simulink model "main__"  (R2013b)
settings: Solver=ode3  StartTime=0.0  StopTime=inf  RelTol=1e-3
undefined symbols (not defined in the file): DiscIntNeverNeededParam, st_, Standard_Devices, UDP_Protocol
libraries: rtwinlib x4
settings Model: SimulationMode=external  ExtModeTrigDuration=1000001  BufferReuse=off  Creator=Nabeel  LastModifiedBy=Nabeel Ahmad
settings SolverCC: AutoInsertRateTranBlk=on
settings DataIOCC: LimitDataPoints=off  SaveOutput=off  SaveTime=off
settings OptimizationCC: OptimizeBlockIOStorage=off  BufferReuse=off  ExpressionFolding=off  LocalBlockOutputs=off
settings DebuggingCC: StateNameClashWarn=warning
settings HardwareCC: ProdIntDivRoundTo=Zero  ProdEndianess=LittleEndian  ProdHWDeviceType=Generic->32-bit x86 compatible
settings RTWCC: SystemTargetFile=rtwin.tlc  TemplateMakefile=rtwin.tmf  Description=Real-Time Windows Target  ProcessScript=rtwin_make_rtw_hook  RTWCompilerOptimization=On
settings CodeAppCC: MaxIdLength=95
settings RTWinTargetCC: TargetLibSuffix=_rtwin.lib  TargetPreCompLibLocation=C:\Program Files\MATLAB\R2013b\toolbox\rtw\targets\rtwin\lib\win64  CodeReplacementLibrary=ANSI_C  RTWinDir=C:/PROGRA~1/MATLAB/R2013b/toolbox/rtw/targets/rtwin  TargetArch=win64

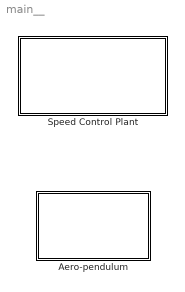
== system main__ ==
  Aero-pendulum : Subsystem
  Speed Control Plant : Subsystem

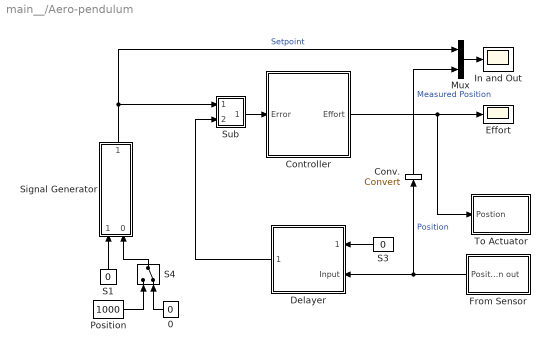
== system main__/Aero-pendulum ==
  0 : Constant  Value=0
  Controller : Subsystem
  Conv. : DataTypeConversion
  Delayer : Subsystem
  Effort : Scope
      settings: TimeRange=100  YMin=33.5  YMax=33.5  SaveName=ScopeData4
  From Sensor : Subsystem
  In and Out : Scope
      settings: ShowLegends=on  TimeRange=40  YMin=-90  YMax=90  SaveName=ScopeData5
  Mux : Mux  Inputs=2
  Position : Constant  Value=1000
  S1 : Constant  Value=0
  S3 : Constant  Value=0
  S4 : ManualSwitch  CurrentSetting=0
  Signal Generator : Subsystem
  Sub : Subsystem
  To Actuator : Subsystem
  wires:
  Delayer/1(Output) -> Sub/2(F)
  Controller/1(Effort) -> To Actuator/1(Postion), Effort/1
  Signal Generator/1(Set Point) -> Mux/1, Sub/1(S)  "Setpoint"
  S3/1 -> Delayer/1(Setting)
  Conv./1 -> Mux/2  "Measured Position"
  Mux/1 -> In and Out/1
  Sub/1(E) -> Controller/1(Error)
  From Sensor/1(Position out) -> Delayer/2(Input), Conv./1  "Position"
  Position/1 -> S4/1
  S4/1 -> Signal Generator/2(0)
  0/1 -> S4/2
  S1/1 -> Signal Generator/1(Setting)

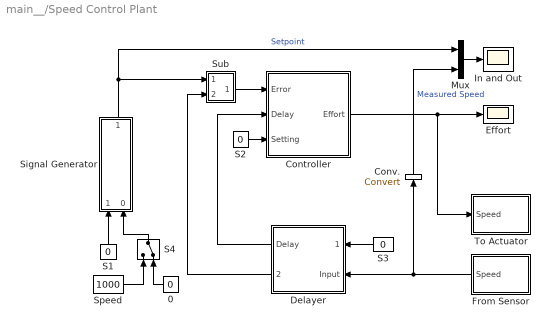
== system main__/Speed Control Plant ==
  0 : Constant  Value=0
  Controller : Subsystem
  Conv. : DataTypeConversion
  Delayer : Subsystem
  Effort : Scope
      settings: TimeRange=100  YMin=-2136.75  YMax=-1933.25
  From Sensor : Subsystem
  In and Out : Scope
      settings: ShowLegends=on  TimeRange=60  YMin=-500  YMax=2100
  Mux : Mux  Inputs=2
  S1 : Constant  Value=0
  S2 : Constant  Value=0
  S3 : Constant  Value=0
  S4 : ManualSwitch  CurrentSetting=0
  Signal Generator : Subsystem
  Speed : Constant  Value=1000
  Sub : Subsystem
  To Actuator : Subsystem
  wires:
  Conv./1 -> Mux/2  "Measured Speed"
  Controller/1(Effort) -> To Actuator/1(Speed), Effort/1
  S2/1 -> Controller/3(Setting)
  Speed/1 -> S4/1
  S4/1 -> Signal Generator/2(0)
  0/1 -> S4/2
  From Sensor/1(Speed) -> Delayer/2(Input), Conv./1
  Signal Generator/1(Set Point) -> Sub/1(S), Mux/1  "Setpoint"
  S1/1 -> Signal Generator/1(Setting)
  Mux/1 -> In and Out/1
  Sub/1(E) -> Controller/1(Error)
  Delayer/1(Delay) -> Controller/2(Delay)
  S3/1 -> Delayer/1(Setting)
  Delayer/2(Output) -> Sub/2(F)

== system main__/Aero-pendulum/Controller ==
  Error : Inport
  I : Constant  Value=.4
  P : Constant  Value=.15
  PI Controller : Subsystem
  Trigger : Constant  Value=0
  Effort : Outport
  wires:
  Trigger/1 -> PI Controller/4(Reset)
  I/1 -> PI Controller/3(I)
  P/1 -> PI Controller/2(P)
  Error/1 -> PI Controller/1(Error)
  PI Controller/1(Effort) -> Effort/1  "Effort"

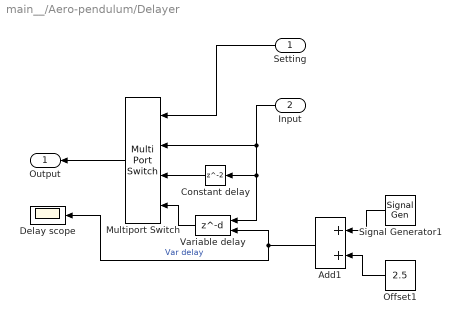
== system main__/Aero-pendulum/Delayer ==
  Setting : Inport
  Input : Inport  Port=2
  Add1 : Sum  OutDataTypeStr=uint8
  Constant delay : Delay  InitialCondition=0  SampleTime=st_
  Delay scope : Scope
      settings: TimeRange=100  YMin=0  SaveName=ScopeData2
  Multiport Switch : MultiPortSwitch  DataPortOrder=Zero-based contiguous
  Offset1 : Constant  Value=2.5
  Signal Generator1 : SignalGenerator  WaveForm=sawtooth  Amplitude=2.5  Frequency=.01
  Variable delay : Delay  DelayLengthSource=Input port  InitialCondition=0  SampleTime=st_
      settings: InputPortMap=u0,p1
  Output : Outport
  wires:
  Setting/1 -> Multiport Switch/1
  Variable delay/1 -> Multiport Switch/4
  Multiport Switch/1 -> Output/1
  Signal Generator1/1 -> Add1/1
  Add1/1 -> Delay scope/1, Variable delay/2  "Var delay"
  Offset1/1 -> Add1/2
  Input/1 -> Multiport Switch/2, Variable delay/1, Constant delay/1
  Constant delay/1 -> Multiport Switch/3

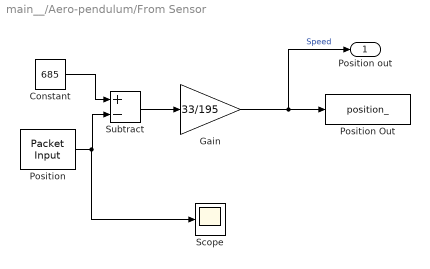
== system main__/Aero-pendulum/From Sensor ==
  Constant : Constant  Value=685
  Gain : Gain  Gain=33/195
  Position : rtwinlib/Packet Input  SampleTime=st_  MaxMissedTicks=10  ShowMissedTicks=off  YieldWhenWaiting=off  DrvName=Standard_Devices/UDP_Protocol  DrvAddress=12349  DrvOptions=[3232235531 43210]  PacketSize=2  DataTypes='int16'  ShowReady=off  ShowError=off  PacketID=1  ByteOrder=1  ShowTimestamp=off
      settings: AttributesFormatString=Standard Devices\nUDP Protocol [303Dh]
  Position Out : ToWorkspace  VariableName=position_  SampleTime=st_  SaveFormat=Structure With Time
  Scope : Scope
      settings: YMin=0  YMax=850  SaveName=ScopeData3
  Subtract : Sum  Inputs=+-
  Position out : Outport
  wires:
  Gain/1 -> Position Out/1, Position out/1  "Speed"
  Subtract/1 -> Gain/1
  Constant/1 -> Subtract/1
  Position/1 -> Scope/1, Subtract/2

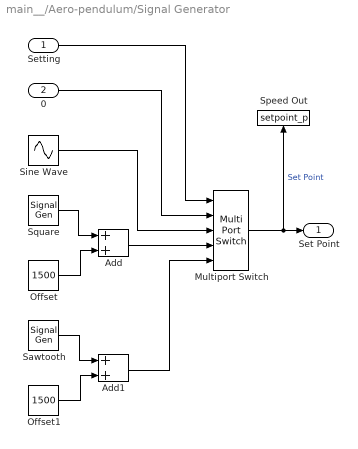
== system main__/Aero-pendulum/Signal Generator ==
  Setting : Inport
  0 : Inport  Port=2
  Add : Sum
  Add1 : Sum
  Multiport Switch : MultiPortSwitch  DataPortOrder=Zero-based contiguous  Inputs=4
  Offset : Constant  Value=1500
  Offset1 : Constant  Value=1500
  Sawtooth : SignalGenerator  WaveForm=square  Amplitude=400  Frequency=.2
  Sine Wave : Sin  Amplitude=7  Bias=15  Frequency=.2  SampleTime=0
  Speed Out : ToWorkspace  VariableName=setpoint_p  SampleTime=st_  SaveFormat=Structure With Time
  Square : SignalGenerator  WaveForm=sawtooth  Amplitude=400  Frequency=.2
  Set Point : Outport
  wires:
  Offset/1 -> Add/2
  Multiport Switch/1 -> Speed Out/1, Set Point/1  "Set Point"
  Setting/1 -> Multiport Switch/1
  Add/1 -> Multiport Switch/4
  0/1 -> Multiport Switch/2
  Sine Wave/1 -> Multiport Switch/3
  Square/1 -> Add/1
  Offset1/1 -> Add1/2
  Add1/1 -> Multiport Switch/5
  Sawtooth/1 -> Add1/1

== system main__/Aero-pendulum/Sub ==
  S : Inport
  F : Inport  Port=2
  Constant : Constant  Value=0
  Manual Switch : ManualSwitch  CurrentSetting=0
  Sum : Sum  Inputs=|+-
  E : Outport
  wires:
  Sum/1 -> E/1
  S/1 -> Sum/1
  Constant/1 -> Manual Switch/1
  F/1 -> Manual Switch/2
  Manual Switch/1 -> Sum/2

== system main__/Aero-pendulum/To Actuator ==
  Postion : Inport
  Position Out : ToWorkspace  VariableName=effort_p  SampleTime=st_  SaveFormat=Structure With Time
  Position Set Point : rtwinlib/Packet Output  SampleTime=st_  MaxMissedTicks=10  ShowMissedTicks=off  YieldWhenWaiting=off  DrvName=Standard_Devices/UDP_Protocol  DrvAddress=12351  DrvOptions=[3232235531 43210]  PacketSize=2  DataTypes='int16'  ShowReady=off  ShowError=off  PacketID=1  ByteOrder=1  InitialValue=[]  FinalValue=[]
      settings: AttributesFormatString=Standard Devices\nUDP Protocol [303Fh]
  Position to PWM duty : Gain  Gain=255/33
  wires:
  Postion/1 -> Position to PWM duty/1, Position Out/1
  Position to PWM duty/1 -> Position Set Point/1

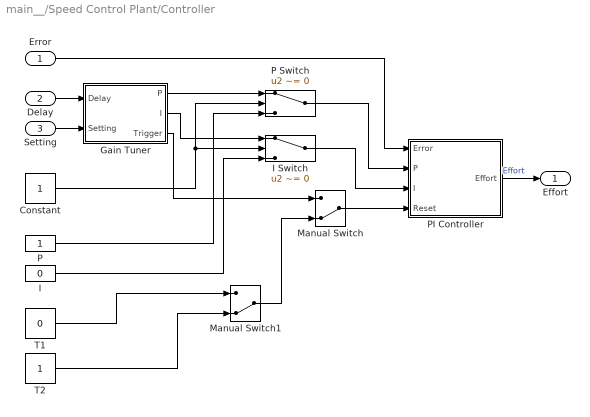
== system main__/Speed Control Plant/Controller ==
  Error : Inport
  Delay : Inport  Port=2
  Setting : Inport  Port=3
  Constant : Constant
  Gain Tuner : MATLAB Function  TreatAsAtomicUnit=on
  I : Constant  Value=0
  I Switch : Switch  Criteria=u2 ~= 0
  Manual Switch : ManualSwitch  CurrentSetting=0
  Manual Switch1 : ManualSwitch  CurrentSetting=0
  P : Constant
  P Switch : Switch  Criteria=u2 ~= 0
  PI Controller : Subsystem
  T1 : Constant  Value=0
  T2 : Constant
  Effort : Outport
  wires:
  Error/1 -> PI Controller/1(Error)
  PI Controller/1(Effort) -> Effort/1  "Effort"
  Delay/1 -> Gain Tuner/1(Delay)
  Setting/1 -> Gain Tuner/2(Setting)
  Constant/1 -> P Switch/2, I Switch/2
  P Switch/1 -> PI Controller/2(P)
  I Switch/1 -> PI Controller/3(I)
  P/1 -> P Switch/3
  I/1 -> I Switch/3
  Gain Tuner/1(P) -> P Switch/1
  Gain Tuner/2(I) -> I Switch/1
  Manual Switch/1 -> PI Controller/4(Reset)
  Gain Tuner/3(Trigger) -> Manual Switch/1
  T1/1 -> Manual Switch1/1
  T2/1 -> Manual Switch1/2
  Manual Switch1/1 -> Manual Switch/2

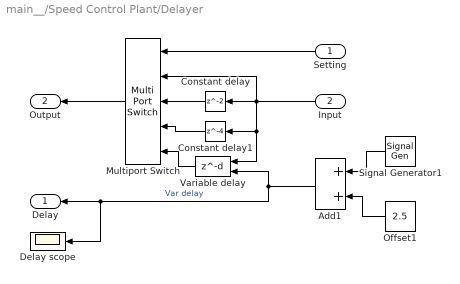
== system main__/Speed Control Plant/Delayer ==
  Setting : Inport
  Input : Inport  Port=2
  Add1 : Sum  OutDataTypeStr=uint8
  Constant delay : Delay  InitialCondition=0  SampleTime=.1
  Constant delay1 : Delay  DelayLength=4  InitialCondition=0  SampleTime=.1
  Delay scope : Scope
      settings: TimeRange=100  YMin=0  SaveName=ScopeData2
  Multiport Switch : MultiPortSwitch  DataPortOrder=Zero-based contiguous  Inputs=4
  Offset1 : Constant  Value=2.5
  Signal Generator1 : SignalGenerator  WaveForm=sawtooth  Amplitude=2.5  Frequency=.01
  Variable delay : Delay  DelayLengthSource=Input port  InitialCondition=0  SampleTime=.1
      settings: InputPortMap=u0,p1
  Delay : Outport
  Output : Outport  Port=2
  wires:
  Setting/1 -> Multiport Switch/1
  Variable delay/1 -> Multiport Switch/5
  Multiport Switch/1 -> Output/1
  Signal Generator1/1 -> Add1/1
  Add1/1 -> Delay scope/1, Delay/1, Variable delay/2  "Var delay"
  Offset1/1 -> Add1/2
  Input/1 -> Multiport Switch/2, Variable delay/1, Constant delay1/1, Constant delay/1
  Constant delay/1 -> Multiport Switch/3
  Constant delay1/1 -> Multiport Switch/4

== system main__/Speed Control Plant/From Sensor ==
  Count to Speed : Gain  Gain=1000/95
  Speed Out : ToWorkspace  VariableName=speed_  SampleTime=.1  SaveFormat=Structure With Time
  Speed_ : rtwinlib/Packet Input  SampleTime=.1  MaxMissedTicks=10  ShowMissedTicks=off  YieldWhenWaiting=off  DrvName=Standard_Devices/UDP_Protocol  DrvAddress=12347  DrvOptions=[3232235530 43210]  PacketSize=2  DataTypes='int16'  ShowReady=off  ShowError=off  PacketID=1  ByteOrder=1  ShowTimestamp=off
      settings: AttributesFormatString=Standard Devices\nUDP Protocol [303Bh]
  Speed : Outport
  wires:
  Count to Speed/1 -> Speed Out/1, Speed/1  "Speed"
  Speed_/1 -> Count to Speed/1

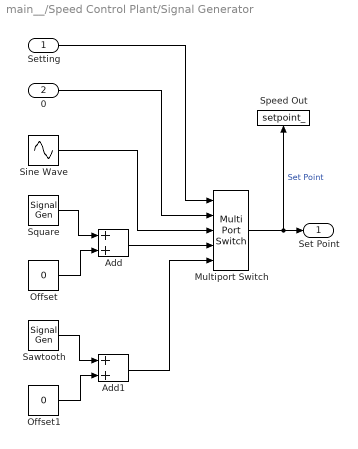
== system main__/Speed Control Plant/Signal Generator ==
  Setting : Inport
  0 : Inport  Port=2
  Add : Sum
  Add1 : Sum
  Multiport Switch : MultiPortSwitch  DataPortOrder=Zero-based contiguous  Inputs=4
  Offset : Constant  Value=0
  Offset1 : Constant  Value=0
  Sawtooth : SignalGenerator  WaveForm=square  Amplitude=400  Frequency=.2
  Sine Wave : Sin  Amplitude=400  Bias=1000  Frequency=.2  SampleTime=0
  Speed Out : ToWorkspace  VariableName=setpoint_  SampleTime=.1  SaveFormat=Structure With Time
  Square : SignalGenerator  WaveForm=sawtooth  Amplitude=400  Frequency=.2
  Set Point : Outport
  wires:
  Offset/1 -> Add/2
  Multiport Switch/1 -> Speed Out/1, Set Point/1  "Set Point"
  Setting/1 -> Multiport Switch/1
  Add/1 -> Multiport Switch/4
  0/1 -> Multiport Switch/2
  Sine Wave/1 -> Multiport Switch/3
  Square/1 -> Add/1
  Offset1/1 -> Add1/2
  Add1/1 -> Multiport Switch/5
  Sawtooth/1 -> Add1/1

== system main__/Speed Control Plant/Sub ==
  S : Inport
  F : Inport  Port=2
  Constant : Constant  Value=0
  Manual Switch : ManualSwitch  CurrentSetting=0
  Sum : Sum  Inputs=|+-
  E : Outport
  wires:
  Sum/1 -> E/1
  S/1 -> Sum/1
  Constant/1 -> Manual Switch/1
  F/1 -> Manual Switch/2
  Manual Switch/1 -> Sum/2

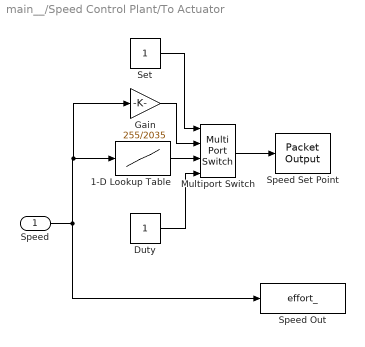
== system main__/Speed Control Plant/To Actuator ==
  Speed : Inport
  1-D Lookup Table : Lookup_n-D  NumberOfTableDimensions=1  BreakpointsForDimension1=[-2035 -1950 -1770 -1585 -1405 -1220 -1045 -870 -690 -500 -320 -230 -140 -60 -0.1 0 60 140 230 320 500 690 870 1045 1220 1405 1585 1770 1950 2035]  Table=[-255 -240 -220 -200 -180 -160 -140 -120 -100 -80 -60 -50 -40 -30 -25 25 30 40 50 60 80 100 120 140 160 180 200 220 240 255]  ExtrapMethod=Clip  InternalRulePriority=Speed  RndMeth=Simplest  InputSameDT=on
  Duty : Constant
  Gain : Gain  Gain=255/2035
  Multiport Switch : MultiPortSwitch  DataPortOrder=Zero-based contiguous
  Set : Constant
  Speed Out : ToWorkspace  VariableName=effort_  SampleTime=.1  SaveFormat=Structure With Time
  Speed Set Point : rtwinlib/Packet Output  SampleTime=.1  MaxMissedTicks=10  ShowMissedTicks=off  YieldWhenWaiting=off  DrvName=Standard_Devices/UDP_Protocol  DrvAddress=12345  DrvOptions=[3232235530 43210]  PacketSize=2  DataTypes='int16'  ShowReady=off  ShowError=off  PacketID=1  ByteOrder=1  InitialValue=[]  FinalValue=[]
      settings: AttributesFormatString=Standard Devices\nUDP Protocol [3039h]
  wires:
  Multiport Switch/1 -> Speed Set Point/1
  1-D Lookup Table/1 -> Multiport Switch/3
  Duty/1 -> Multiport Switch/4
  Gain/1 -> Multiport Switch/2
  Speed/1 -> Gain/1, 1-D Lookup Table/1, Speed Out/1
  Set/1 -> Multiport Switch/1

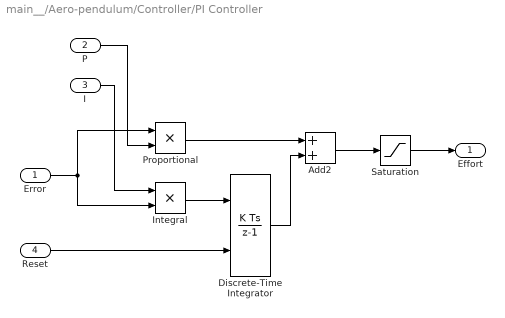
== system main__/Aero-pendulum/Controller/PI Controller ==
  Error : Inport
  P : Inport  Port=2
  I : Inport  Port=3
  Reset : Inport  Port=4
  Add2 : Sum  SampleTime=st_
  Discrete-Time Integrator : DiscreteIntegrator  ExternalReset=falling  SampleTime=st_  ICPrevOutput=DiscIntNeverNeededParam  ICPrevScaledInput=DiscIntNeverNeededParam
  Integral : Product  SampleTime=st_
  Proportional : Product  SampleTime=st_
  Saturation : Saturate  UpperLimit=33  LowerLimit=-33  SampleTime=st_
  Effort : Outport
  wires:
  Proportional/1 -> Add2/1
  Add2/1 -> Saturation/1
  Discrete-Time Integrator/1 -> Add2/2
  P/1 -> Proportional/2
  Integral/1 -> Discrete-Time Integrator/1
  I/1 -> Integral/1
  Error/1 -> Integral/2, Proportional/1
  Saturation/1 -> Effort/1
  Reset/1 -> Discrete-Time Integrator/2

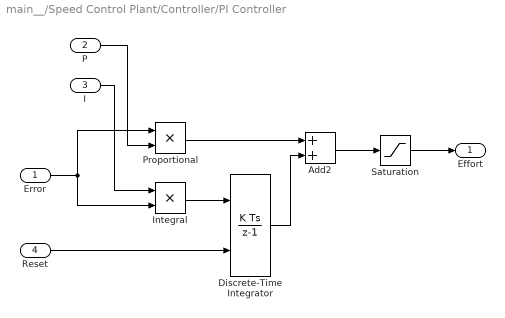
== system main__/Speed Control Plant/Controller/PI Controller ==
  Error : Inport
  P : Inport  Port=2
  I : Inport  Port=3
  Reset : Inport  Port=4
  Add2 : Sum  SampleTime=.1
  Discrete-Time Integrator : DiscreteIntegrator  ExternalReset=falling  SampleTime=.1  ICPrevOutput=DiscIntNeverNeededParam  ICPrevScaledInput=DiscIntNeverNeededParam
  Integral : Product  SampleTime=.1
  Proportional : Product  SampleTime=.1
  Saturation : Saturate  UpperLimit=2035  LowerLimit=-2035  SampleTime=.1
  Effort : Outport
  wires:
  Proportional/1 -> Add2/1
  Add2/1 -> Saturation/1
  Discrete-Time Integrator/1 -> Add2/2
  P/1 -> Proportional/2
  Integral/1 -> Discrete-Time Integrator/1
  I/1 -> Integral/1
  Error/1 -> Integral/2, Proportional/1
  Saturation/1 -> Effort/1
  Reset/1 -> Discrete-Time Integrator/2

== matlab function main__/Speed Control Plant/Controller/Gain Tuner ==
  settings: updateMethod=DISCRETE  sampleTime=0.1
  data: Delay input; P output; I output; Trigger output [-1..1]; Setting input
function [P, I, Trigger]= fcn(Delay, Setting)
%#codegen

persistent setting;
if isempty(setting)
    setting=0;
end

if Setting==0
    % % For un-tuned controller
    P = 0.427580000000000;
    I = 2.179900000000000;
    Trigger = 0;
    
else
    % For auto-tuned controller
    if Delay==0
        P = 0.427580000000000;
        I = 2.179900000000000;
    elseif Delay>0 && Delay<=1
        P = 0.365940000000000;
        I = 1.654100000000000;
    elseif Delay>1 && Delay<=2
        P = 0.383940000000000;
        I = 1.403900000000000;
    elseif Delay>2 && Delay<=3
        P = 0.324080000000000;
        I = 1.160800000000000;
    elseif Delay>3 && Delay<=4
        P = 0.352910000000000;
        I = 1.027200000000000;
    else
        P = 0.332100000000000;
        I = 0.896710000000000;
    end
end

if Setting==2
    % Reset trigger singal. Should be commented for un-tuned controller.
    if setting~=double(ceil(Delay))
        Trigger=-1;
        setting=double(ceil(Delay));
    else
        Trigger=1;
    end
else
    Trigger=0;
end
